simulink model "WaveModulation"  (R2024a)
settings: Solver=VariableStepAuto  StartTime=0.0  StopTime=1  RelTol=1e-3
settings Model: Creator=BIDO  LastModifiedBy=BIDO

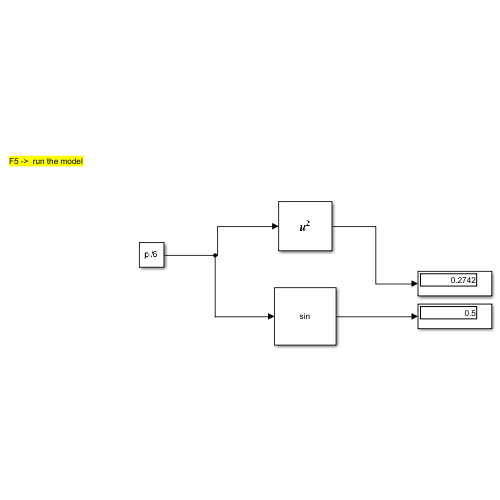
[thumbnail: Simulink's stored preview of the top-level diagram]
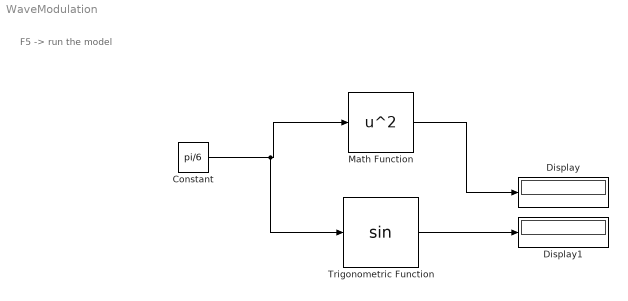
== system WaveModulation ==
  note: F5 -> run the model
  Constant : Constant  Value=pi/6
  Display : Display
  Display1 : Display
  Math Function : Math  Operator=square
  Trigonometric Function : Trigonometry
  wires:
  Constant/1 -> Trigonometric Function/1, Math Function/1
  Math Function/1 -> Display/1
  Trigonometric Function/1 -> Display1/1
